simulink model "tp5_5_recepteur_corrige_simple"  (R2023a)
settings: Solver=VariableStepDiscrete  StartTime=0.0  StopTime=inf  RelTol=1e-3
PreLoadFcn:
  | T_s_short=160e-6;
  | N=36;
  | N_IFFT=64;
  | T_e = T_s_short/N_IFFT;
  | f_e=1/T_e;
  | 
  | 
  | %% nombre d'éléments nuls à ajouter au vecteur X, resp avant et après les N ss porteuses actives
  | Z_d=ceil((N_IFFT-N)/2);
  | Z_u=floor((N_IFFT-N)/2);
  | 
  | %% taille du préfixe cyclique et temps symbole rallongé
  | v=8;
  | T_s=(N_IFFT+v)*T_e;
  | 
  | %% pilotes
  | r=0.25;
  | 
  | %% la trame
  | t=10;
  | T_t=t*T_s;
  | 
  | %% le canal
  | delays=[0 ceil((200e-9)/T_e)*T_e ceil((500e-9)/T_e)*T_e];
  | gains = [0 -3 -6];
  | 
  | %% le codage binaire du message
  | capa_symbole = N*(1-r)*2;
  | str='coucou';
  | message=double(dec2bin(str,8)=='1');% zeros(6-strlength(str),8)];
  | assert(capa_symbole > numel(message), 'message trop long');
  | message_pad=capa_symbole-numel(message);
InitFcn:
  | T_s_short=160e-6;
  | N=36;
  | N_IFFT=64;
  | T_e = T_s_short/N_IFFT;
  | f_e=1/T_e;
  | 
  | 
  | %% nombre d'éléments nuls à ajouter au vecteur X, resp avant et après les N ss porteuses actives
  | Z_d=ceil((N_IFFT-N)/2);
  | Z_u=floor((N_IFFT-N)/2);
  | 
  | %% taille du préfixe cyclique et temps symbole rallongé
  | v=8;
  | T_s=(N_IFFT+v)*T_e;
  | 
  | %% pilotes
  | r=0.25;
  | 
  | %% la trame
  | t=10;
  | T_t=t*T_s;
  | 
  | %% le canal
  | delays=[0 ceil((200e-9)/T_e)*T_e ceil((500e-9)/T_e)*T_e];
  | gains = [0 -3 -6];
  | 
  | %% le codage binaire du message
  | capa_symbole = N*(1-r)*2;
  | str='coucou';
  | message=double(dec2bin(str,8)=='1');% zeros(6-strlength(str),8)];
  | assert(capa_symbole > numel(message), 'message trop long');
  | message_pad=capa_symbole-numel(message);
undefined symbols (not defined in the file or in its folder): designMultirateFIR, jsin, magnitude
libraries: dspindex x8, simulink x1, dspxfrm3 x1, dspmlti4 x1, commdigbbndpm3 x1, sdrrlib x1, dspsigops x1
settings Model: SimulationMode=accelerator  Creator=speychet  LastModifiedBy=pjoseph
settings SolverCC: AlgebraicLoopSolver=TrustRegion
settings DataIOCC: LimitDataPoints=on  SaveOutput=off  SaveTime=off
settings OptimizationCC: BooleanDataType=off  DefaultParameterBehavior=Inlined  LocalBlockOutputs=off  LifeSpan=inf
settings DebuggingCC: AlgebraicLoopMsg=error  SingleTaskRateTransMsg=error  UnconnectedInputMsg=warning  UnconnectedOutputMsg=warning  UnconnectedLineMsg=warning  AllowSymbolicDim=off  SFUnexpectedBacktrackingDiag=warning  SFNoUnconditionalDefaultTransitionDiag=warning  SFExecutionAtInitializationDiag=none  ArithmeticOperatorsInVariantConditions=warning
settings ModelReferenceCC: EnableRefExpFcnMdlSchedulingChecks=on
settings SFSimCC: SimUseLocalCustomCode=off  CustomCodeUndefinedFunction=UseInterfaceOnly
settings RTWCC: RTWUseLocalCustomCode=off
settings CodeAppCC: StateflowObjectComments=on
settings GRTTargetCC: TargetLangStandard=C89/C90 (ANSI)
settings ConfigComp: CovMetricSettings=dw  CovSaveCumulativeToWorkspaceVar=on  CovSaveSingleToWorkspaceVar=on  CovExternalEMLEnable=off  CovSFcnEnable=off

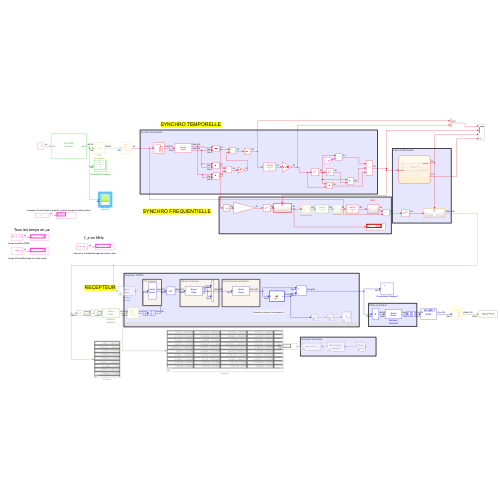
[thumbnail: Simulink's stored preview of the top-level diagram]
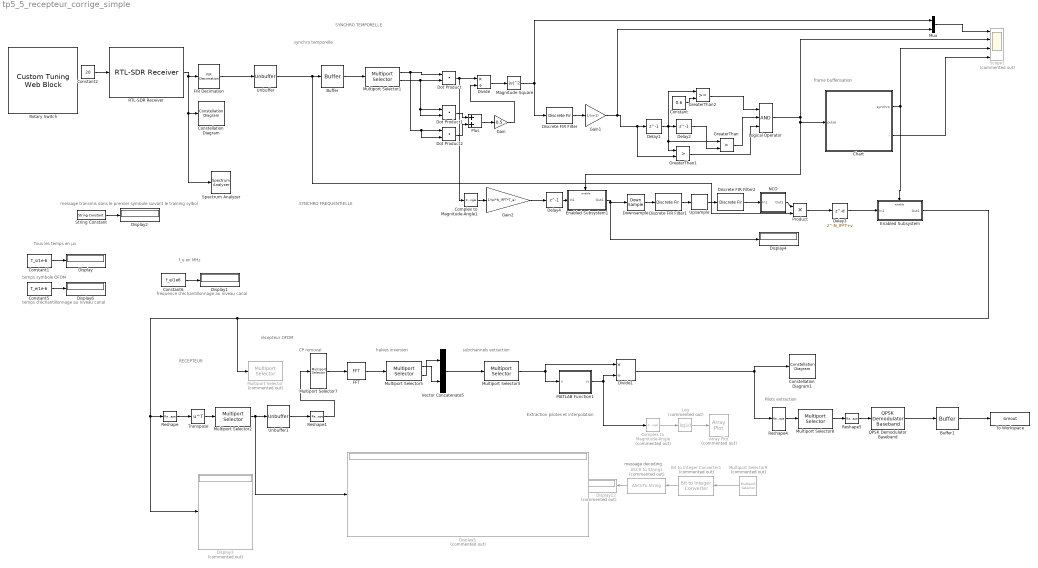
== system tp5_5_recepteur_corrige_simple ==
  note: frame bufferisation
  note: message decoding
  note: Pilots extraction
  note: synchro temporelle
  note: message transmis dans le premier symbole suivant le training sylbol
  note: SYNCHRO TEMPORELLE
  note: halves inversion
  note: subchannels extraction
  note: récepteur OFDM
  note: CP removal
  note: Extraction pilotes et interpolation
  note: temps d'échantillonnage au niveau canal
  note: fréquence d'échantillonnage au niveau canal
  note: f_e en MHz
  note: temps symbole OFDM
  note: Tous les temps en µs
  note: RECEPTEUR
  note: SYNCHRO FREQUENTIELLE
  ASCII to String1 : ASCIIToString  Commented=on
  Array Plot : ArrayPlot  Commented=on  WindowPosition=[601.000000,98.000000,800.000000,500.000000,]  ScopeFrameLocation=window  YLimits=[-0.4671,-0.0335]  ShowLegend=on
  Bit to Integer Converter1 : simulink/Logic and Bit Operations/Bit to Integer Converter  Commented=on  nbits=8  bitOrder=MSB first  signedOutputValues=Unsigned  outDtype=uint8  outDtypeSigned=Inherit via internal rule
      settings: LibrarySourceBlock=|
      | commutil2/Bit to Integer
      | Converter
  Buffer : Buffer  N=N_IFFT  V=N_IFFT-1  OutputFrames=off
  Buffer1 : Buffer  N=N*(1-r)*2*(t-1)  OutputFrames=off
  Chart : Stateflow chart  TreatAsAtomicUnit=on
  Complex to Magnitude-Angle : ComplexToMagnitudeAngle  Commented=on  Output=Magnitude
  Complex to Magnitude-Angle1 : ComplexToMagnitudeAngle  Output=Angle
  Constant : Constant  Value=0.6
  Constant1 : Constant  Value=T_s/1e-6
  Constant2 : Constant  Value=20
  Constant5 : Constant  Value=T_e/1e-6
  Constant6 : Constant  Value=f_e/1e6
  Constellation Diagram : ConstellationDiagram  WindowPosition=[364.000000,153.000000,600.000000,600.000000,]  Visible=on  ScopeFrameLocation=window
  Constellation Diagram1 : ConstellationDiagram  WindowPosition=[963.000000,198.000000,461.000000,428.000000,]  Visible=on  ScopeFrameLocation=window  SymbolsToDisplaySource=Property  SymbolsToDisplay=200  XLimits=[-1.375,1.375]  YLimits=[-1.375,1.375]  DefaultConfigurationName=comm.scopes.ConstellationDiagramBlockCfg
  Delay1 : Delay  DelayLength=1
  Delay2 : Delay  DelayLength=1
  Delay3 : Delay  DelayLength=N_IFFT+v
  Delay4 : Delay  DelayLength=1
  Discrete FIR Filter : DiscreteFir  Coefficients=ones(1,v+1)
  Discrete FIR Filter1 : DiscreteFir  Coefficients=ones(1,100)*1/100
  Discrete FIR Filter2 : DiscreteFir  Coefficients=ones(1,(N_IFFT+v)*t)
  Display{,1..2,4,6} (5 alike) : Display
  Display12 : Display  Commented=on
  Display3 : Display  Commented=on
  Display5 : Display  Commented=on
  Divide : Product  Inputs=*/
  Divide1 : Product  Inputs=*/
  Dot Product : DotProduct  OutDataTypeStr=Inherit: Inherit via internal rule
  Dot Product1 : DotProduct  OutDataTypeStr=Inherit: Inherit via internal rule
  Dot Product2 : DotProduct  OutDataTypeStr=Inherit: Inherit via internal rule
  Downsample : DownSample  N=(N_IFFT+v)*t  RateOptions=Allow multirate processing
  Enabled Subsystem : Subsystem  TreatAsAtomicUnit=on
      settings: LibrarySourceBlock=|
      | hdlsllib/Ports &
      | Subsystems/Enabled
      | Subsystem
  Enabled Subsystem1 : Subsystem  TreatAsAtomicUnit=on
      settings: LibrarySourceBlock=|
      | hdlsllib/Ports &
      | Subsystems/Enabled
      | Subsystem
  FFT : dspxfrm3/FFT  FFTImplementation=Auto  CompMethod=Table lookup  TableOpt=NEW  TableOptActive=Speed  BitRevOrder=off  Normalize=off  InheritFFTLength=on  FFTLength=64  WrapInput=on  roundingMode=Floor  overflowMode=off  firstCoeffDataTypeStr=Inherit: Same word length as input  firstCoeffLastDataTypeStr=Inherit: Same word length as input  outputMin=[]  outputMax=[]
  FIR Decimation : dspmlti4/FIR Decimation  FilterSource=Auto  h=designMultirateFIR(1,2)  D=4  filtStruct=Direct form  FilterObject=FDECIM  InputProcessing=Columns as channels (frame based)  framing=Allow multirate processing  AllowArbitraryInputLength=off  inputOffset=0  outputBufInitCond=0  roundingMode=Floor  overflowMode=off  firstCoeffDataTypeStr=Inherit: Same word length as input  firstCoeffMin=[]  firstCoeffMax=[]  firstCoeffLastDataTypeStr=Inherit: Same word length as input  outputDataTypeStr=Inherit: Same as accumulator  outputMin=[]  outputMax=[]  outputLastDataTypeStr=Inherit: Same as accumulator
      settings: LibrarySourceBlock=|
      | dsphdlsupportfiltering/FIR
      | Decimation
  Gain : Gain  Gain=0.5
  Gain1 : Gain  Gain=1/(v+1)
  Gain2 : Gain  Gain=1/(pi*N_IFFT*T_e)
  GreaterThan : RelationalOperator  Operator=>  OutDataTypeStr=boolean  RndMeth=Simplest  InputSameDT=off
  GreaterThan1 : RelationalOperator  Operator=>  OutDataTypeStr=boolean  RndMeth=Simplest  InputSameDT=off
  GreaterThan2 : RelationalOperator  OutDataTypeStr=boolean  RndMeth=Simplest  InputSameDT=off
  Log : Math  Commented=on  Operator=log10
  Logical Operator : Logic  Inputs=3  AllPortsSameDT=off  OutDataTypeStr=boolean
  MATLAB Function1 : MATLAB Function  TreatAsAtomicUnit=on
  Magnitude Square : Math  Operator=magnitude^2  SignedPower=on  RndMeth=Zero
  Multiport Selector : dspindex/Multiport Selector  Commented=on  rowsOrCols=Rows  idxCellArray={ 2*(N_IFFT+v)+1:3*(N_IFFT+v) }  idxErrMode=Clip Index
      settings: LibrarySourceBlock=|
      | dsphdlsupportsigmgmt/Multiport
      | Selector
  Multiport Selector1 : dspindex/Multiport Selector  rowsOrCols=Rows  idxCellArray={ [1:N_IFFT/2], [N_IFFT/2+1:N_IFFT] }  idxErrMode=Clip Index
  Multiport Selector2 : dspindex/Multiport Selector  rowsOrCols=Rows  idxCellArray={ 2:t }  idxErrMode=Clip Index
      settings: LibrarySourceBlock=|
      | dsphdlsupportsigmgmt/Multiport
      | Selector
  Multiport Selector3 : dspindex/Multiport Selector  rowsOrCols=Rows  idxCellArray={ Z_d+1:N_IFFT-Z_u}  idxErrMode=Clip Index
  Multiport Selector5 : dspindex/Multiport Selector  rowsOrCols=Rows  idxCellArray={ [1:N_IFFT/2], [N_IFFT/2+1:N_IFFT] }  idxErrMode=Clip Index
  Multiport Selector7 : dspindex/Multiport Selector  rowsOrCols=Rows  idxCellArray={[v+1:N_IFFT+v]}  idxErrMode=Clip Index
  Multiport Selector8 : dspindex/Multiport Selector  rowsOrCols=Rows  idxCellArray=1:(1-r)/r  idxErrMode=Clip Index
      settings: LibrarySourceBlock=|
      | dsphdlsupportsigmgmt/Multiport
      | Selector
  Multiport Selector9 : dspindex/Multiport Selector  Commented=on  rowsOrCols=Rows  idxCellArray=1:numel(message)  idxErrMode=Clip Index
  Mux : Mux  Inputs=2
  "NCO " : Subsystem
  Plus : Sum
  Product : Product
  QPSK Demodulator Baseband : commdigbbndpm3/QPSK Demodulator Baseband  OutType=Bit  DecType=Hard decision  VarSource=Dialog  Variance=1  Dec=Gray  Ph=pi/4  outDtype1=Inherit via internal rule  outDtype2=Inherit via internal rule  derotateFactorWordLen=16  derotateFactorDataTypeStr=Inherit: Same word length as input  derotateFactorLastDataTypeStr=Inherit: Same word length as input
      settings: LibrarySourceBlock=|
      | commhdldigbbndpm/QPSK
      | Demodulator
      | Baseband
  RTL-SDR Receiver : sdrrlib/RTL-SDR Receiver  IPAddress=0  CenterFrequencySource=Dialog  CenterFrequency=433.5e6  GainSource=Input port  Gain=0  ADCRate=1.6e6  FrequencyCorrection=0  LostSamplesOutputPort=off  LatencyOutputPort=off  OutputDataType=double  FrameLength=72*4  EnableBurstMode=on  NumFramesInBurst=1000  sobjType=sdrr.internal.SDRRTLReceiverSL  dataUDPPort=-1  ctrlUDPPort=-1  subDeviceList=nosubdev  sdrBlockType=SDRBlockTypeSLT.SDRRxBlock  requester=UNUSED_BY_SFCN  sdrExecutionMode=SDRExecutionModeSLT.ExecModeHW  BypassUserLogic=off  DecimatorSelect=DDC decimator  SourceSelect=RF data  SineAmplitude=16000  EnableInternalClock=off  BypassIQBalance=off  IFBandwidth=40e6  ADCRateSource=Dialog  IntermediateFrequency=0  DecimationFactorSource=Dialog  DecimationFactor=512  RFFrequencyIsTunable=logical(0)  SampleTime=(72*4)/(1.6e6)  IFBandwidthSource=Dialog  SineFrequency=30000  BypassDCBlockingFilter=off  IntermediateFrequencySource=Dialog  IQBalanceCoefficients=64  SkipAllHardwareResetAndInitialization=off  EnableIQCalibrationTable=on  CacheIQCalibrationTable=off  EnableOffsetTuning=off  EnableRTLAGC=off  EnableTestMode=off  EnableTunerAGC=off  FrequencyCorrectionSource=Dialog  NumMLBuffers=128  NumUSBBuffers=16  RTLCrystalFrequency=28800000  TunerCrystalFrequency=28800000
  Reshape : Reshape  OutputDimensionality=Customize  OutputDimensions=[N_IFFT+v,t]
  Reshape1 : Reshape  OutputDimensionality=Column vector (2-D)
  Reshape4 : Reshape  OutputDimensionality=Customize  OutputDimensions=[1/r,N*r]
  Reshape5 : Reshape  OutputDimensionality=Column vector (2-D)
  Rotary Switch : CustomTuningWebBlock  LabelPosition=Hide  ShowInitialText=on  Configuration="{\"components\":[{\"name\":\"RotarySwitchComponent\",\"settings\":{\"arcAngle\":300,\"arcAngleOffset\":120,\"handle\":{\"size\":[150,150],\"src\":\"data:image\\/svg+xml;base64,PHN2ZyBpZD0iTGF5ZXJfMSIgZGF0YS1uYW1lPSJMYXllciAxIiB4bWxucz0iaHR0cDovL3d3dy53My5vcmcvMjAwMC9zdmciIHhtbG5zOnhsaW5rPSJodHRwOi8vd3d3LnczLm9yZy8xOTk5L3hsaW5rIiB2aWV3Qm94PSIwIDAgMTIxIDEyMSI+PGRlZnM+PHN0eWxlPi5jbHMtMXtmaWxsOnVybCgjbGluZWFyLWdyYWRpZW50KTt9LmNscy0yLC5jbHMtM3tmaWxsOiNkMWQxZDE7fS5jbHMtM3tzdHJva2U6I2I3YjdiNztzdHJva2UtbWl0ZXJsaW1pdDoxMDtzdHJva2Utd2lkdGg6MC4yNXB4O30uY2xzLTR7ZmlsbDojZjMwMDAwO30uY2xzLTV7ZmlsbDojZjIxNzY3O308L3N0eWxlPjxsaW5lYXJHcmFkaWVudCBpZD0ibGluZWFyLWdyYWRpZW50IiB4MT0iNjAuNSIgeTE9IjEyMC41IiB4Mj0iNjAuNSIgeTI9IjAuNSIgZ3JhZGllbnRVbml0cz0idXNlclNwYWNlT25Vc2UiPjxzdG9wIG9mZnNldD0iMCIgc3RvcC1jb2xvcj0iI2QxZDFkMSIvPjxzdG9wIG9mZnNldD0iMC4xIiBzdG9wLWNvbG9yPSIjY2VjZWNlIi8+PHN0b3Agb2Zmc2V0PSIwLjE5IiBzdG9wLWNvbG9yPSIjYzNjM2MzIi8+PHN0b3Agb2Zmc2V0PSIwLjI4IiBzdG9wLWNvbG9yPSIjYjFiMWIxIi8+PHN0b3Agb2Zmc2V0PSIwLjM2IiBzdG9wLWNvbG9yPSIjOTg5ODk4Ii8+PHN0b3Agb2Zmc2V0PSIwLjQ0IiBzdG9wLWNvbG9yPSIjNzg3ODc4Ii8+PHN0b3Agb2Zmc2V0PSIwLjQ2IiBzdG9wLWNvbG9yPSIjNmI2YjZiIi8+PHN0b3Agb2Zmc2V0PSIwLjU0IiBzdG9wLWNvbG9yPSIjNmI2YjZiIi8+PHN0b3Agb2Zmc2V0PSIwLjU2IiBzdG9wLWNvbG9yPSIjNzY3Njc2Ii8+PHN0b3Agb2Zmc2V0PSIwLjY0IiBzdG9wLWNvbG9yPSIjOTc5Nzk3Ii8+PHN0b3Agb2Zmc2V0PSIwLjcyIiBzdG9wLWNvbG9yPSIjYjBiMGIwIi8+PHN0b3Agb2Zmc2V0PSIwLjgxIiBzdG9wLWNvbG9yPSIjYzNjM2MzIi8+PHN0b3Agb2Zmc2V0PSIwLjkiIHN0b3AtY29sb3I9IiNjZGNkY2QiLz48c3RvcCBvZmZzZXQ9IjEiIHN0b3AtY29sb3I9IiNkMWQxZDEiLz48L2xpbmVhckdyYWRpZW50PjwvZGVmcz48Y2lyY2xlIGNsYXNzPSJjbHMtMSIgY3g9IjYwLjUiIGN5PSI2MC41IiByPSI2MCIvPjxwYXRoIGNsYXNzPSJjbHMtMiIgZD0iTTYwLjUsMUE1OS41LDU5LjUsMCwxLDEsMSw2MC41LDU5LjU3LDU5LjU3LDAsMCwxLDYwLjUsMW0wLTFBNjAuNSw2MC41LDAsMSwwLDEyMSw2MC41LDYwLjUsNjAuNSwwLDAsMCw2MC41LDBaIi8+PHJlY3QgY2xhc3M9ImNscy0zIiB4PSIwLjUiIHk9IjUxLjUiIHdpZHRoPSIxMjAiIGhlaWdodD0iMTgiIHJ4PSIzLjA0Ii8+PHJlY3QgY2xhc3M9ImNscy00IiB4PSI1Ljc1IiB5PSI1OC43NSIgd2lkdGg9IjE2IiBoZWlnaHQ9IjMiLz48cGF0aCBjbGFzcz0iY2xzLTUiIGQ9Ik0yMS4yNSw1OS4yNXYyaC0xNXYtMmgxNW0xLTFoLTE3djRoMTd2LTRaIi8+PC9zdmc+\"},\"handleOffset\":[0,0],\"handleOrientation\":180,\"handlePosition\":[0,0,1,1],\"handleSize\":{\"height\":0.5,\"width\":0.5},\"labelRadius\":0.36,\"position\":[0,0,1,1],\"states\":[{\"Label\":{\"color\":[0,0,0,1],\"icon\":{\"size\":[0,0],\"src\":[],\"srcOrientation\":\"Right\"},\"iconPlacement\":\"left\",\"opacity\":1,\"position\":[0.7345552884615385,0.6796274038461538],\"show\":true,\"text\":{\"content\":\"10\",\"font\":\"Helvetica\",\"fontSize\":24}},\"Value\":10},{\"Label\":{\"color\":[0,0,0,1],\"icon\":{\"size\":[0,0],\"src\":[],\"srcOrientation\":\"Right\"},\"iconPlacement\":\"left\",\"opacity\":1,\"position\":[0.35757211538461536,0.7603966346153846],\"show\":true,\"text\":{\"content\":\"20\",\"font\":\"Helvetica\",\"fontSize\":24}},\"Value\":20},{\"Label\":{\"color\":[0,0,0,1],\"icon\":{\"size\":[0,0],\"src\":[],\"srcOrientation\":\"Right\"},\"iconPlacement\":\"left\",\"opacity\":1,\"position\":[0.09603365384615385,0.46033653846153844],\"show\":true,\"text\":{\"content\":\"30\",\"font\":\"Helvetica\",\"fontSize\":24}},\"Value\":30},{\"Label\":{\"color\":[0,0,0,1],\"icon\":{\"size\":[0,0],\"src\":[],\"srcOrientation\":\"Right\"},\"iconPlacement\":\"left\",\"opacity\":1,\"position\":[0.36532451923076925,0.1180889423076923],\"show\":true,\"text\":{\"content\":\"40\",\"font\":\"Helvetica\",\"fontSize\":24}},\"Value\":40},{\"Label\":{\"color\":[0,0,0,1],\"icon\":{\"size\":[0,0],\"src\":[],\"srcOrientation\":\"Right\"},\"iconPlacement\":\"left\",\"opacity\":1,\"position\":[0.7191706730769231,0.19501201923076922],\"show\":true,\"text\":{\"content\":\"50\",\"font\":\"Helvetica\",\"fontSize\":24}},\"Value\":50}],\"tickRadius\":0.32}},{\"name\":\"BackgroundImageComponent\",\"settings\":{\"image\":{\"size\":[155,150],\"src\":\"data:image\\/svg+xml;base64,PD94bWwgdmVyc2lvbj0iMS4wIiBlbmNvZGluZz0idXRmLTgiPz4NCjwhLS0gR2VuZXJhdG9yOiBBZG9iZSBJbGx1c3RyYXRvciAyNS4wLjAsIFNWRyBFeHBvcnQgUGx1Zy1JbiAuIFNWRyBWZXJzaW9uOiA2LjAwIEJ1aWxkIDApICAtLT4NCjxzdmcgdmVyc2lvbj0iMS4xIg0KCSBpZD0iTGF5ZXJfMl8xXyIgeG1sbnM6Y2M9Imh0dHA6Ly9jcmVhdGl2ZWNvbW1vbnMub3JnL25zIyIgeG1sbnM6ZGM9Imh0dHA6Ly9wdXJsLm9yZy9kYy9lbGVtZW50cy8xLjEvIiB4bWxuczppbmtzY2FwZT0iaHR0cDovL3d3dy5pbmtzY2FwZS5vcmcv ...(+4184 chars)\",\"srcOrientation\":\"Right\"},\"position\":[0,0,1,1],\"scaleMode\":\"0\"}},{\"name\":\"ForegroundImageComponent\",\"settings\":{\"image\":{\"size\":[0,0],\"src\":\"default\",\"srcOrientation\":[]},\"isForeground\":1,\"position\":[0,0,1,1],\"scaleMode\":\"0\"}}],\"settings\":{\"BindingType\":\"param\",\"backgroundColor\":[0,0,255,\"1\"],\"backgroundOffset\":1,\"fixedAspectRatio\":\"on\",\"image\":{\"size\":[150,150],\"src\":\"data:image\\/svg+xml;base64,PD94bWwgdmVyc2lvbj0iMS4wIiBlbmNvZGluZz0iVVRGLTgiIHN0YW5kYWxvbmU9Im5vIj8+CjwhLS0gR2VuZXJhdG9yOiBBZG9iZSBJbGx1c3RyYXRvciAxOS4yLjEsIFNWRyBFeHBvcnQgUGx1Zy1JbiAuIFNWRyBWZXJzaW9uOiA2LjAwIEJ1aWxkIDApICAtLT4KCjxzdmcKICAgeG1sbnM6ZGM9Imh0dHA6Ly9wdXJsLm9yZy9kYy9lbGVtZW50cy8xLjEvIgogICB4bWxuczpjYz0iaHR0cDovL2NyZWF0aXZlY29tbW9ucy5vcmcvbnMjIgogICB4bWxuczpyZGY9Imh0dHA6Ly93d3cudzMub3JnLzE5OTkvMDIvMjItcmRmLXN5bnRh ...(+9660 chars)\"},\"showBackgroundColor\":false,\"variant\":\"rotarySwitch\",\"version\":\"R2023a\"},\"type\":\"RotarySwitch\"}"
  Scope1 : Scope  Commented=on  NumInputPorts=4
  Spectrum Analyzer : SpectrumAnalyzer  WindowPosition=[263.000000,176.000000,800.000000,500.000000,]  Visible=on  ScopeFrameLocation=window  Span=1600000  StartFrequency=-800000  StopFrequency=800000  YLimits=[-58.66994507,0.19600502]  ColorLimits=[-80 20]
  String Constant : StringConstant  String=str
  To Workspace : ToWorkspace  VariableName=simout  SaveFormat=Timeseries  SampleTime=-1
  Transpose : Math  Operator=transpose
  Unbuffer : Unbuffer
  Unbuffer1 : Unbuffer
  Upsample : dspsigops/Upsample  FactorSource=Dialog parameter  N=(N_IFFT+v)*t  Nmax=16  phase=0  RateOptions=Allow multirate processing  ic=0  mode=Unused parameter value
      settings: LibrarySourceBlock=dsphdlsupportsigops/Upsample
  Vector Concatenate5 : Concatenate
  wires:
  String Constant/1 -> Display2/1
  Buffer/1 -> Multiport Selector1/1
  Discrete FIR Filter/1 -> Gain1/1
  Multiport Selector1/2 -> Dot Product1/2, Dot Product1/1, Dot Product/2
  Dot Product/1 -> Divide/1, Complex to Magnitude-Angle1/1
  Divide/1 -> Magnitude Square/1
  Dot Product2/1 -> Plus/2
  Dot Product1/1 -> Plus/1
  Multiport Selector1/1 -> Dot Product2/2, Dot Product2/1, Dot Product/1
  Gain/1 -> Divide/2
  Plus/1 -> Gain/1
  Delay1/1 -> GreaterThan1/1, GreaterThan/1, GreaterThan2/1, Delay2/1
  Constant/1 -> GreaterThan2/2
  Delay2/1 -> GreaterThan/2
  GreaterThan2/1 -> Logical Operator/1
  GreaterThan/1 -> Logical Operator/2
  GreaterThan1/1 -> Logical Operator/3
  Magnitude Square/1 -> Discrete FIR Filter/1, Mux/1
  Gain1/1 -> Mux/2, GreaterThan1/2, Delay1/1
  Multiport Selector5/1 -> Vector Concatenate5/2
  Multiport Selector7/1 -> FFT/1
  Multiport Selector3/1 -> Divide1/1, MATLAB Function1/1(Y)
  Enabled Subsystem/1(Out1) -> Reshape/1, Display3/1, Multiport Selector/1
  Vector Concatenate5/1 -> Multiport Selector3/1
  Complex to Magnitude-Angle/1 -> Log/1
  Log/1 -> Array Plot/1
  FFT/1 -> Multiport Selector5/1
  Multiport Selector5/2 -> Vector Concatenate5/1
  Divide1/1 -> Constellation Diagram1/1, Reshape4/1
  MATLAB Function1/1(H) -> Complex to Magnitude-Angle/1, Divide1/2
  Delay3/1 -> Enabled Subsystem/1(In1)
  Chart/1(synchro) -> Enabled Subsystem/Enable, Scope1/3
  ASCII to String1/1 -> Display12/1
  Bit to Integer Converter1/1 -> ASCII to String1/1
  Reshape4/1 -> Multiport Selector8/1
  Multiport Selector8/1 -> Reshape5/1
  Reshape5/1 -> QPSK Demodulator Baseband/1
  Multiport Selector9/1 -> Bit to Integer Converter1/1
  Constant6/1 -> Display1/1
  Constant1/1 -> Display/1
  Constant5/1 -> Display6/1
  Complex to Magnitude-Angle1/1 -> Gain2/1
  Gain2/1 -> Delay4/1
  Delay4/1 -> Enabled Subsystem1/1(In1)
  Unbuffer/1 -> Buffer/1, Product/2
  Downsample/1 -> Discrete FIR Filter1/1
  Discrete FIR Filter1/1 -> Upsample/1
  Upsample/1 -> Discrete FIR Filter2/1
  Discrete FIR Filter2/1 -> "NCO "/1(In1)
  Logical Operator/1 -> Scope1/2, Enabled Subsystem1/Enable, Chart/1(pulse)
  "NCO "/1(Out1) -> Product/1
  Product/1 -> Delay3/1
  FIR Decimation/1 -> Unbuffer/1
  RTL-SDR Receiver/1 -> Spectrum Analyzer/1, Constellation Diagram/1, FIR Decimation/1
  Constant2/1 -> RTL-SDR Receiver/1
  Mux/1 -> Scope1/1
  Chart/2(i) -> Scope1/4
  Enabled Subsystem1/1(Out1) -> Downsample/1, Display4/1
  QPSK Demodulator Baseband/1 -> Buffer1/1
  Buffer1/1 -> To Workspace/1
  Reshape/1 -> Transpose/1
  Unbuffer1/1 -> Reshape1/1
  Reshape1/1 -> Multiport Selector7/1
  Transpose/1 -> Multiport Selector2/1
  Multiport Selector2/1 -> Display5/1, Unbuffer1/1

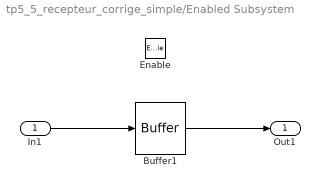
== system tp5_5_recepteur_corrige_simple/Enabled Subsystem ==
  In1 : Inport
  Enable : EnablePort  StatesWhenEnabling=reset
  Buffer1 : Buffer  N=(N_IFFT+v)*t  OutputFrames=off
  Out1 : Outport
  wires:
  In1/1 -> Buffer1/1
  Buffer1/1 -> Out1/1

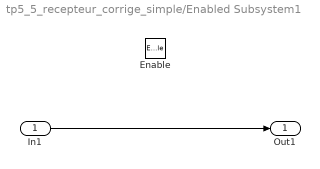
== system tp5_5_recepteur_corrige_simple/Enabled Subsystem1 ==
  In1 : Inport
  Enable : EnablePort
  Out1 : Outport
  wires:
  In1/1 -> Out1/1

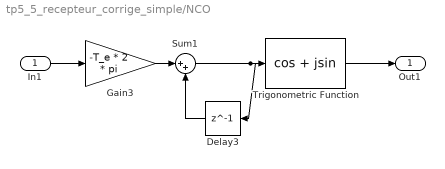
== system tp5_5_recepteur_corrige_simple/NCO  ==
  In1 : Inport
  Delay3 : Delay  DelayLength=1  InitialCondition=0
  Gain3 : Gain  Gain=-T_e * 2 * pi
  Sum1 : Sum  Inputs=|++
  Trigonometric Function : Trigonometry  Operator=cos + jsin
  Out1 : Outport  VectorParamsAs1DForOutWhenUnconnected=off
  wires:
  Gain3/1 -> Sum1/1
  Delay3/1 -> Sum1/2
  Sum1/1 -> Delay3/1, Trigonometric Function/1
  In1/1 -> Gain3/1
  Trigonometric Function/1 -> Out1/1

== matlab function tp5_5_recepteur_corrige_simple/MATLAB Function1 ==
  data: Y input; H output; N parameter; r parameter
function H = fcn(Y, N, r)

H=Y;              %initialisation de H avec Y; ceci remplit les pilotes (les autres positions doivent être écrasées

H(1:1/r-1) = Y(1/r)*(ones(1,1/r-1));  % les 1/r-1 premières positions sont égales au premier pilote

prev_pilot=Y(1/r);  % initialisation pour la boucle

for i=1/r : 1/r : N-1/r+1
  pilot=Y(i+1/r);
  pente = (pilot-prev_pilot)/(1/r);
    for j=1:1/r-1
        
        H(i+j)=prev_pilot+pente*j;
    end
   prev_pilot=pilot;
end

== stateflow chart tp5_5_recepteur_corrige_simple/Chart ==
  state SEARCH
    entry : synchro=0;
    state PULSE_FOUND
    state NEXT_PULSE_SHOULD_BE_CLOSE
      entry : i=4;
      during:
      i=i-1;
    state WAIT_FOR_PULSE
    SEARCH.PULSE_FOUND -> SEARCH.PULSE_FOUND [order 1] : [pulse==1]
    SEARCH.PULSE_FOUND -> SEARCH.NEXT_PULSE_SHOULD_BE_CLOSE [order 2] : after(N_IFFT*t+v*t-2, tick)
    WAIT_FOR_PULSE -> SEARCH.PULSE_FOUND : [pulse==1]
    SEARCH.NEXT_PULSE_SHOULD_BE_CLOSE -> WAIT_FOR_PULSE [order 1] : [i==0]
  state LOCK
    entry : synchro=1;
    state NEXT_PULSE_SHOULD_BE_CLOSE
      entry : i=4;
      during:
      i=i-1;
      note: ]
    state PULSE_FOUND
    LOCK.PULSE_FOUND -> LOCK.NEXT_PULSE_SHOULD_BE_CLOSE : after(N_IFFT*t+v*t-2, tick)
    LOCK.NEXT_PULSE_SHOULD_BE_CLOSE -> LOCK.PULSE_FOUND [order 1] : [pulse==1]
  (default) -> WAIT_FOR_PULSE
  LOCK.NEXT_PULSE_SHOULD_BE_CLOSE -> WAIT_FOR_PULSE [order 2] : [i==0]
  SEARCH.NEXT_PULSE_SHOULD_BE_CLOSE -> LOCK.PULSE_FOUND [order 2] : [pulse==1]
  data: synchro output; pulse input; v parameter; N_IFFT parameter; t parameter double; i output int8 size=1
